simulink model "transient_fault_using_simulink"  (R2022a)
settings: Solver=VariableStepAuto  StartTime=0.0  StopTime=0.5  RelTol=1e-3
settings Model: Creator=agnav  LastModifiedBy=agnav

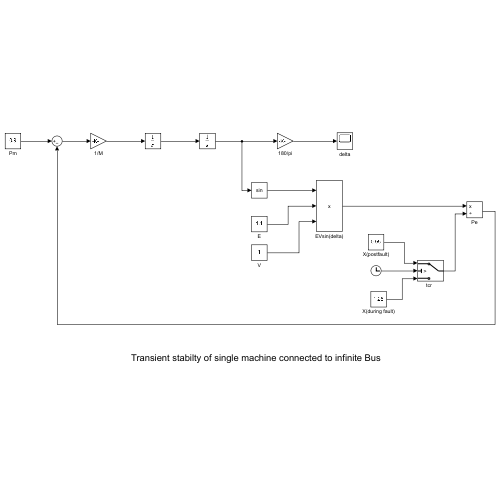
[thumbnail: Simulink's stored preview of the top-level diagram]
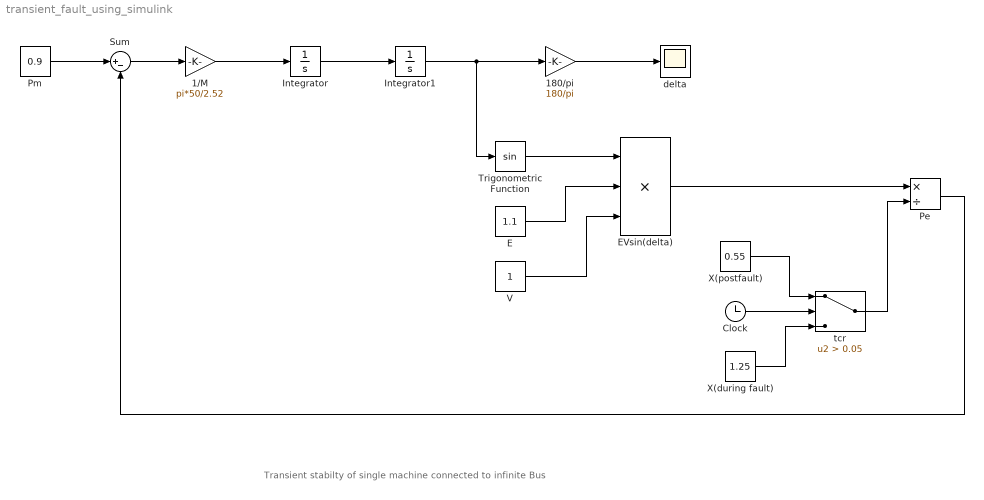
== system transient_fault_using_simulink ==
  note: Transient stabilty of single machine connected to infinite Bus
  1/M : Gain  Gain=pi*50/2.52
  180/pi : Gain  Gain=180/pi
  Clock : Clock
  E : Constant  Value=1.1
  EVsin(delta) : Product  Inputs=3
  Integrator : Integrator  InitialCondition=21.64*pi/180
  Integrator1 : Integrator  InitialCondition=21.64*pi/180
  Pe : Product  Inputs=*/
  Pm : Constant  Value=0.9
  Sum : Sum  Inputs=|+-
  Trigonometric Function : Trigonometry
  V : Constant
  X(during fault) : Constant  Value=1.25
  X(postfault) : Constant  Value=0.55
  delta : Scope
  "tcr  " : Switch  Criteria=u2 > Threshold  Threshold=0.05  SaturateOnIntegerOverflow=off  InputSameDT=off
  wires:
  Integrator/1 -> Integrator1/1
  1/M/1 -> Integrator/1
  Integrator1/1 -> Trigonometric Function/1, 180/pi/1
  Trigonometric Function/1 -> EVsin(delta)/1
  E/1 -> EVsin(delta)/2
  V/1 -> EVsin(delta)/3
  X(postfault)/1 -> "tcr  "/1
  X(during fault)/1 -> "tcr  "/3
  Clock/1 -> "tcr  "/2
  EVsin(delta)/1 -> Pe/1
  "tcr  "/1 -> Pe/2
  Pm/1 -> Sum/1
  Sum/1 -> 1/M/1
  Pe/1 -> Sum/2
  180/pi/1 -> delta/1
